simulink library "MainLibrary"  (R2022b)
settings: Solver=VariableStepAuto  StartTime=0.0  StopTime=10.0  RelTol=1e-3
undefined symbols (not defined in the file or in its folder): A, B, C, G, g0, g00, g00d, g0d, H, K, Kd, Ke, Ked, T, WO
libraries: $bdroot x14
settings Model: Creator=cotti  LastModifiedBy=cotti

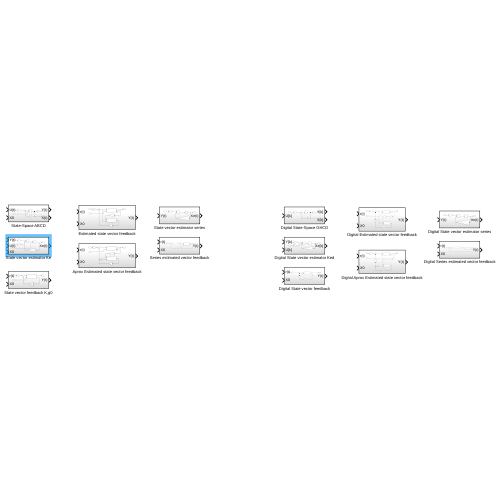
[thumbnail: Simulink's stored preview of the top-level diagram]
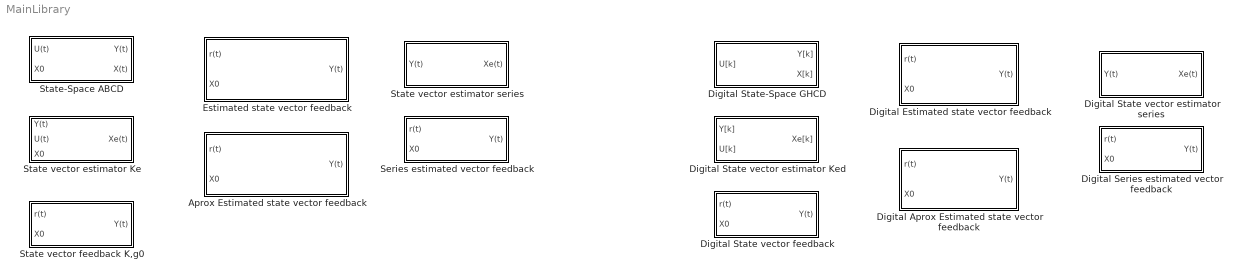
== system MainLibrary ==
  Aprox Estimated state vector feedback : Subsystem
  Digital Aprox Estimated state vector feedback : Subsystem
  Digital Estimated state vector feedback : Subsystem
  Digital Series estimated vector feedback : Subsystem
  Digital State vector estimator Ked : Subsystem
  Digital State vector estimator series : Subsystem
  Digital State vector feedback : Subsystem
  Digital State-Space GHCD : Subsystem
  Estimated state vector feedback : Subsystem
  Series estimated vector feedback : Subsystem
  State vector estimator Ke : Subsystem
  State vector estimator series : Subsystem
  State vector feedback K,g0 : Subsystem
  State-Space ABCD : Subsystem

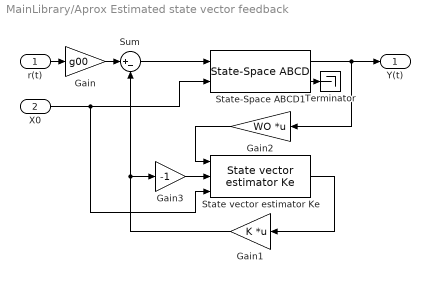
== system MainLibrary/Aprox Estimated state vector feedback ==
  r(t) : Inport
  X0 : Inport  Port=2
  Gain : Gain  Gain=g00
  Gain1 : Gain  Gain=K  Multiplication=Matrix(K*u)
  Gain2 : Gain  Gain=WO  Multiplication=Matrix(K*u)
  Gain3 : Gain  Gain=-1
  State vector estimator Ke : $bdroot/State vector estimator Ke  SystemSampleTime=-1  VariantActivationTime=update diagram  Latency=0  AutoFrameSizeCalculation=off
  State-Space ABCD1 : $bdroot/State-Space ABCD  SystemSampleTime=-1  VariantActivationTime=update diagram  Latency=0  AutoFrameSizeCalculation=off
  Sum : Sum  Inputs=|+-
  Terminator : Terminator
  Y(t) : Outport
  wires:
  Gain/1 -> Sum/1
  Gain1/1 -> Gain3/1, Sum/2
  Sum/1 -> State-Space ABCD1/1
  r(t)/1 -> Gain/1
  State-Space ABCD1/1 -> Gain2/1, Y(t)/1
  State-Space ABCD1/2 -> Terminator/1
  State vector estimator Ke/1 -> Gain1/1
  X0/1 -> State vector estimator Ke/3, State-Space ABCD1/2
  Gain2/1 -> State vector estimator Ke/1
  Gain3/1 -> State vector estimator Ke/2

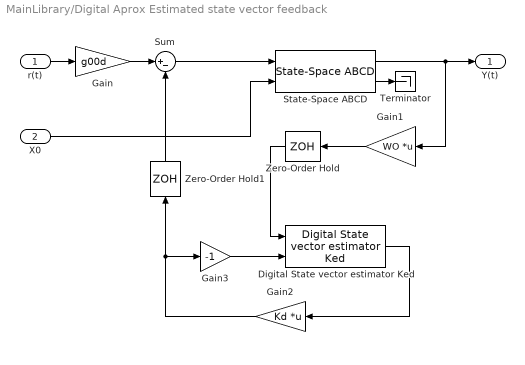
== system MainLibrary/Digital Aprox Estimated state vector feedback ==
  r(t) : Inport
  X0 : Inport  Port=2
  Digital State vector estimator Ked : $bdroot/Digital State vector estimator Ked  SystemSampleTime=-1  VariantActivationTime=update diagram  Latency=0  AutoFrameSizeCalculation=off
  Gain : Gain  Gain=g00d
  Gain1 : Gain  Gain=WO  Multiplication=Matrix(K*u)
  Gain2 : Gain  Gain=Kd  Multiplication=Matrix(K*u)
  Gain3 : Gain  Gain=-1
  State-Space ABCD : $bdroot/State-Space ABCD  SystemSampleTime=-1  VariantActivationTime=update diagram  Latency=0  AutoFrameSizeCalculation=off
  Sum : Sum  Inputs=|+-
  Terminator : Terminator
  Zero-Order Hold : ZeroOrderHold  SampleTime=T
  Zero-Order Hold1 : ZeroOrderHold  SampleTime=T
  Y(t) : Outport
  wires:
  r(t)/1 -> Gain/1
  Gain/1 -> Sum/1
  State-Space ABCD/2 -> Terminator/1
  State-Space ABCD/1 -> Y(t)/1, Gain1/1
  Gain1/1 -> Zero-Order Hold/1
  X0/1 -> State-Space ABCD/2
  Zero-Order Hold/1 -> Digital State vector estimator Ked/1
  Digital State vector estimator Ked/1 -> Gain2/1
  Gain2/1 -> Gain3/1, Zero-Order Hold1/1
  Zero-Order Hold1/1 -> Sum/2
  Sum/1 -> State-Space ABCD/1
  Gain3/1 -> Digital State vector estimator Ked/2

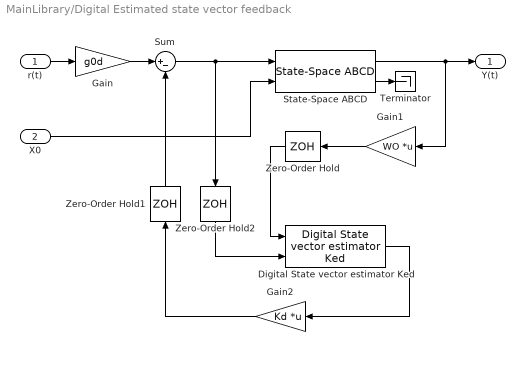
== system MainLibrary/Digital Estimated state vector feedback ==
  r(t) : Inport
  X0 : Inport  Port=2
  Digital State vector estimator Ked : $bdroot/Digital State vector estimator Ked  SystemSampleTime=-1  VariantActivationTime=update diagram  Latency=0  AutoFrameSizeCalculation=off
  Gain : Gain  Gain=g0d
  Gain1 : Gain  Gain=WO  Multiplication=Matrix(K*u)
  Gain2 : Gain  Gain=Kd  Multiplication=Matrix(K*u)
  State-Space ABCD : $bdroot/State-Space ABCD  SystemSampleTime=-1  VariantActivationTime=update diagram  Latency=0  AutoFrameSizeCalculation=off
  Sum : Sum  Inputs=|+-
  Terminator : Terminator
  Zero-Order Hold : ZeroOrderHold  SampleTime=T
  Zero-Order Hold1 : ZeroOrderHold  SampleTime=T
  Zero-Order Hold2 : ZeroOrderHold  SampleTime=T
  Y(t) : Outport
  wires:
  r(t)/1 -> Gain/1
  Gain/1 -> Sum/1
  Sum/1 -> Zero-Order Hold2/1, State-Space ABCD/1
  State-Space ABCD/2 -> Terminator/1
  State-Space ABCD/1 -> Y(t)/1, Gain1/1
  Gain1/1 -> Zero-Order Hold/1
  X0/1 -> State-Space ABCD/2
  Zero-Order Hold/1 -> Digital State vector estimator Ked/1
  Digital State vector estimator Ked/1 -> Gain2/1
  Gain2/1 -> Zero-Order Hold1/1
  Zero-Order Hold1/1 -> Sum/2
  Zero-Order Hold2/1 -> Digital State vector estimator Ked/2

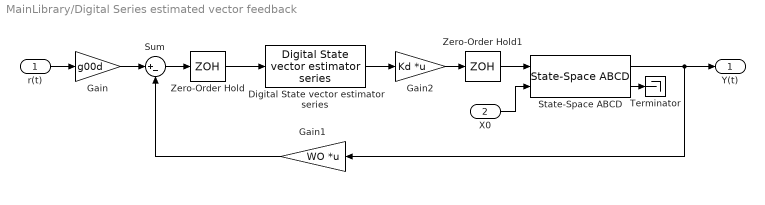
== system MainLibrary/Digital Series estimated vector feedback ==
  r(t) : Inport
  X0 : Inport  Port=2
  Digital State vector estimator series : $bdroot/Digital State vector estimator series  SystemSampleTime=-1  VariantActivationTime=update diagram  Latency=0  AutoFrameSizeCalculation=off
  Gain : Gain  Gain=g00d
  Gain1 : Gain  Gain=WO  Multiplication=Matrix(K*u)
  Gain2 : Gain  Gain=Kd  Multiplication=Matrix(K*u)
  State-Space ABCD : $bdroot/State-Space ABCD  SystemSampleTime=-1  VariantActivationTime=update diagram  Latency=0  AutoFrameSizeCalculation=off
  Sum : Sum  Inputs=|+-
  Terminator : Terminator
  Zero-Order Hold : ZeroOrderHold  SampleTime=-1
  Zero-Order Hold1 : ZeroOrderHold  SampleTime=-1
  Y(t) : Outport
  wires:
  Gain/1 -> Sum/1
  r(t)/1 -> Gain/1
  State-Space ABCD/1 -> Gain1/1, Y(t)/1
  State-Space ABCD/2 -> Terminator/1
  X0/1 -> State-Space ABCD/2
  Digital State vector estimator series/1 -> Gain2/1
  Gain1/1 -> Sum/2
  Gain2/1 -> Zero-Order Hold1/1
  Sum/1 -> Zero-Order Hold/1
  Zero-Order Hold/1 -> Digital State vector estimator series/1
  Zero-Order Hold1/1 -> State-Space ABCD/1

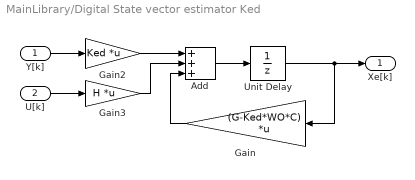
== system MainLibrary/Digital State vector estimator Ked ==
  Y[k] : Inport
  U[k] : Inport  Port=2
  Add : Sum  Inputs=+++
  Gain : Gain  Gain=(G-Ked*WO*C)  Multiplication=Matrix(K*u)
  Gain2 : Gain  Gain=Ked  Multiplication=Matrix(K*u)
  Gain3 : Gain  Gain=H  Multiplication=Matrix(K*u)
  Unit Delay : UnitDelay  SampleTime=T  HasFrameUpgradeWarning=on
  Xe[k] : Outport
  wires:
  Gain2/1 -> Add/1
  Gain3/1 -> Add/2
  U[k]/1 -> Gain3/1
  Gain/1 -> Add/3
  Y[k]/1 -> Gain2/1
  Add/1 -> Unit Delay/1
  Unit Delay/1 -> Gain/1, Xe[k]/1

== system MainLibrary/Digital State vector estimator series ==
  Y(t) : Inport
  Add : Sum
  Gain : Gain  Gain=(G-Ked*WO*C-H*Kd)  Multiplication=Matrix(K*u)
  Gain2 : Gain  Gain=Ked  Multiplication=Matrix(K*u)
  Unit Delay : UnitDelay  SampleTime=T  HasFrameUpgradeWarning=on
  Xe(t) : Outport
  wires:
  Unit Delay/1 -> Xe(t)/1, Gain/1
  Y(t)/1 -> Gain2/1
  Gain2/1 -> Add/1
  Gain/1 -> Add/2
  Add/1 -> Unit Delay/1

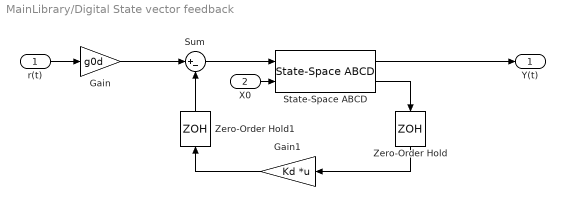
== system MainLibrary/Digital State vector feedback ==
  r(t) : Inport
  X0 : Inport  Port=2
  Gain : Gain  Gain=g0d
  Gain1 : Gain  Gain=Kd  Multiplication=Matrix(K*u)
  State-Space ABCD : $bdroot/State-Space ABCD  SystemSampleTime=-1  VariantActivationTime=update diagram  Latency=0  AutoFrameSizeCalculation=off
  Sum : Sum  Inputs=|+-
  Zero-Order Hold : ZeroOrderHold  SampleTime=T
  Zero-Order Hold1 : ZeroOrderHold  SampleTime=T
  Y(t) : Outport
  wires:
  r(t)/1 -> Gain/1
  Gain/1 -> Sum/1
  Sum/1 -> State-Space ABCD/1
  State-Space ABCD/1 -> Y(t)/1
  State-Space ABCD/2 -> Zero-Order Hold/1
  Zero-Order Hold/1 -> Gain1/1
  Gain1/1 -> Zero-Order Hold1/1
  Zero-Order Hold1/1 -> Sum/2
  X0/1 -> State-Space ABCD/2

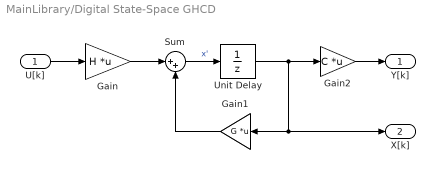
== system MainLibrary/Digital State-Space GHCD ==
  U[k] : Inport
  Gain : Gain  Gain=H  Multiplication=Matrix(K*u)
  Gain1 : Gain  Gain=G  Multiplication=Matrix(K*u)
  Gain2 : Gain  Gain=C  Multiplication=Matrix(K*u)
  Sum : Sum  Inputs=|++
  Unit Delay : UnitDelay  SampleTime=T  HasFrameUpgradeWarning=on
  Y[k] : Outport
  X[k] : Outport  Port=2
  wires:
  Gain2/1 -> Y[k]/1
  Unit Delay/1 -> Gain1/1, X[k]/1, Gain2/1
  Gain/1 -> Sum/1
  Sum/1 -> Unit Delay/1  "x'"
  U[k]/1 -> Gain/1
  Gain1/1 -> Sum/2

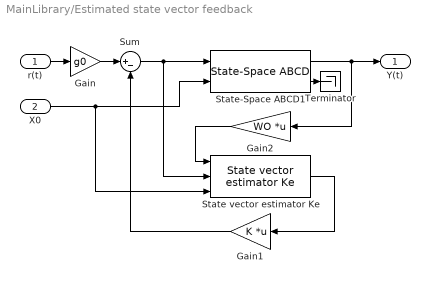
== system MainLibrary/Estimated state vector feedback ==
  r(t) : Inport
  X0 : Inport  Port=2
  Gain : Gain  Gain=g0
  Gain1 : Gain  Gain=K  Multiplication=Matrix(K*u)
  Gain2 : Gain  Gain=WO  Multiplication=Matrix(K*u)
  State vector estimator Ke : $bdroot/State vector estimator Ke  SystemSampleTime=-1  VariantActivationTime=update diagram  Latency=0  AutoFrameSizeCalculation=off
  State-Space ABCD1 : $bdroot/State-Space ABCD  SystemSampleTime=-1  VariantActivationTime=update diagram  Latency=0  AutoFrameSizeCalculation=off
  Sum : Sum  Inputs=|+-
  Terminator : Terminator
  Y(t) : Outport
  wires:
  Gain/1 -> Sum/1
  Gain1/1 -> Sum/2
  Sum/1 -> State vector estimator Ke/2, State-Space ABCD1/1
  r(t)/1 -> Gain/1
  State-Space ABCD1/1 -> Gain2/1, Y(t)/1
  State-Space ABCD1/2 -> Terminator/1
  State vector estimator Ke/1 -> Gain1/1
  X0/1 -> State vector estimator Ke/3, State-Space ABCD1/2
  Gain2/1 -> State vector estimator Ke/1

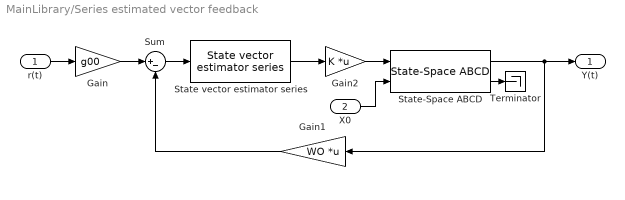
== system MainLibrary/Series estimated vector feedback ==
  r(t) : Inport
  X0 : Inport  Port=2
  Gain : Gain  Gain=g00
  Gain1 : Gain  Gain=WO  Multiplication=Matrix(K*u)
  Gain2 : Gain  Gain=K  Multiplication=Matrix(K*u)
  State vector estimator series : $bdroot/State vector estimator series  SystemSampleTime=-1  VariantActivationTime=update diagram  Latency=0  AutoFrameSizeCalculation=off
  State-Space ABCD : $bdroot/State-Space ABCD  SystemSampleTime=-1  VariantActivationTime=update diagram  Latency=0  AutoFrameSizeCalculation=off
  Sum : Sum  Inputs=|+-
  Terminator : Terminator
  Y(t) : Outport
  wires:
  Gain/1 -> Sum/1
  r(t)/1 -> Gain/1
  State-Space ABCD/1 -> Gain1/1, Y(t)/1
  State-Space ABCD/2 -> Terminator/1
  X0/1 -> State-Space ABCD/2
  State vector estimator series/1 -> Gain2/1
  Sum/1 -> State vector estimator series/1
  Gain1/1 -> Sum/2
  Gain2/1 -> State-Space ABCD/1

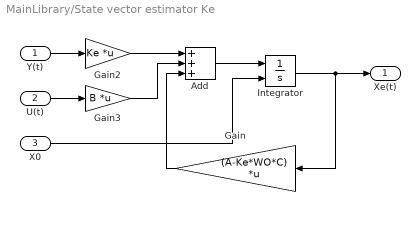
== system MainLibrary/State vector estimator Ke ==
  Y(t) : Inport
  U(t) : Inport  Port=2
  X0 : Inport  Port=3
  Add : Sum  Inputs=+++
  Gain : Gain  Gain=(A-Ke*WO*C)  Multiplication=Matrix(K*u)
  Gain2 : Gain  Gain=Ke  Multiplication=Matrix(K*u)
  Gain3 : Gain  Gain=B  Multiplication=Matrix(K*u)
  Integrator : Integrator  InitialConditionSource=external
  Xe(t) : Outport
  wires:
  Gain/1 -> Add/3
  Integrator/1 -> Gain/1, Xe(t)/1
  U(t)/1 -> Gain3/1
  Y(t)/1 -> Gain2/1
  Add/1 -> Integrator/1
  Gain3/1 -> Add/2
  Gain2/1 -> Add/1
  X0/1 -> Integrator/2

== system MainLibrary/State vector estimator series ==
  Y(t) : Inport
  Add : Sum
  Gain : Gain  Gain=(A-Ke*WO*C-B*K)  Multiplication=Matrix(K*u)
  Gain2 : Gain  Gain=Ke  Multiplication=Matrix(K*u)
  Integrator : Integrator
  Xe(t) : Outport
  wires:
  Integrator/1 -> Xe(t)/1, Gain/1
  Y(t)/1 -> Gain2/1
  Add/1 -> Integrator/1
  Gain2/1 -> Add/1
  Gain/1 -> Add/2

== system MainLibrary/State vector feedback K,g0 ==
  r(t) : Inport
  X0 : Inport  Port=2
  Gain : Gain  Gain=g0
  Gain1 : Gain  Gain=K  Multiplication=Matrix(K*u)
  State-Space ABCD : $bdroot/State-Space ABCD  SystemSampleTime=-1  VariantActivationTime=update diagram  Latency=0  AutoFrameSizeCalculation=off
  Sum : Sum  Inputs=|+-
  Y(t) : Outport
  wires:
  State-Space ABCD/1 -> Y(t)/1
  r(t)/1 -> Gain/1
  Gain/1 -> Sum/1
  Gain1/1 -> Sum/2
  State-Space ABCD/2 -> Gain1/1
  Sum/1 -> State-Space ABCD/1
  X0/1 -> State-Space ABCD/2

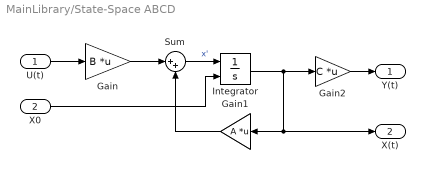
== system MainLibrary/State-Space ABCD ==
  U(t) : Inport
  X0 : Inport  Port=2
  Gain : Gain  Gain=B  Multiplication=Matrix(K*u)
  Gain1 : Gain  Gain=A  Multiplication=Matrix(K*u)
  Gain2 : Gain  Gain=C  Multiplication=Matrix(K*u)
  Integrator : Integrator  InitialConditionSource=external
  Sum : Sum  Inputs=|++
  Y(t) : Outport
  X(t) : Outport  Port=2
  wires:
  Gain1/1 -> Sum/2
  Integrator/1 -> Gain1/1, X(t)/1, Gain2/1
  Sum/1 -> Integrator/1  "x'"
  Gain/1 -> Sum/1
  U(t)/1 -> Gain/1
  Gain2/1 -> Y(t)/1
  X0/1 -> Integrator/2
